simulink model "admittance_control"  (R2024b)
settings: Solver=VariableStepAuto  StartTime=0.0  StopTime=10  FixedStep=0.001  MinStep=1e-5  RelTol=1e-3
undefined symbols (not defined in the file): ddtraj_admittance, dq_i, dtraj_admittance, env1K, env1Normal, env1Origin, Kd_admittance, Kd_motion_control, Kp_admittance, Kp_motion_cotrol, Md_admittance, myRobot, q_i_admittance, traj_admittance, X, Y, Z
libraries: sm_lib x43, matrix_library x7, nesl_utility x4
(part 2 of 2)

== matlab function admittance_control/Subsystem1/h_e norm ==
  data: u input; y output
function y = fcn(u)
    y = norm(u);
end

== matlab function admittance_control/Subsystem1/inside env check ==
  data: u input; y output
function y = fcn(u)
    if u >= 0
        y = 0;
    else 
        y = u;
    end
end

== matlab function admittance_control/Subsystem2/Subsystem2/h_e norm ==
  data: u input; y output
function y = fcn(u)
    y = norm(u);
end

== matlab function admittance_control/Subsystem2/Subsystem2/inside env check ==
  data: u input; y output
function y = fcn(u)
    if u >= 0
        y = 0;
    else 
        y = u;
    end
end

== matlab function admittance_control/Subsystem4/Subsystem2/h_e norm ==
  data: u input; y output
function y = fcn(u)
    y = norm(u);
end
